simulink model "Aufgabe1_sim"  (R2023b)
settings: Solver=VariableStepAuto  StartTime=0.0  StopTime=1  RelTol=1e-3
values from neighbouring files (symbols this model uses):
  ci = 0.01    [Aufgabe1_param.m]
  cy = 1    [Aufgabe1_param.m]
  L = 0.1    [Aufgabe1_param.m]
  m = 10e-3    (= 0.01)    [Aufgabe1_param.m]
  R = 5    [Aufgabe1_param.m]
settings Model: Creator=rouven  LastModifiedBy=rouven

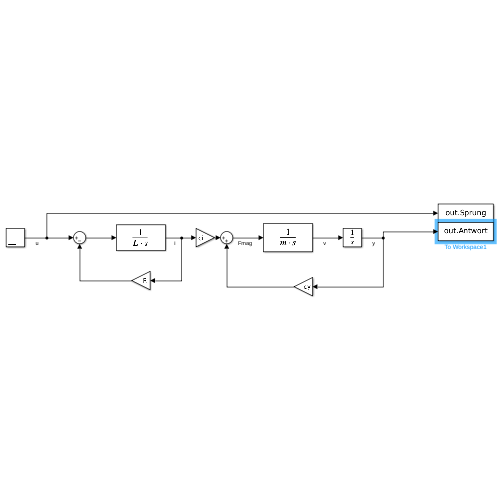
[thumbnail: Simulink's stored preview of the top-level diagram]
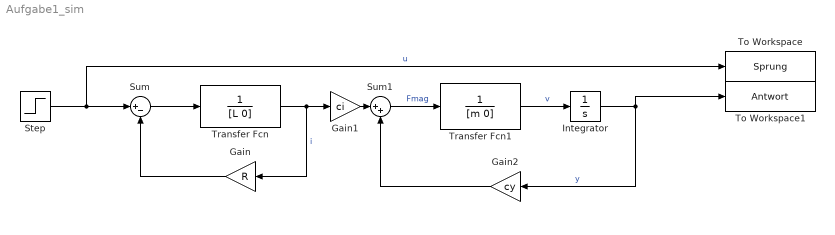
== system Aufgabe1_sim ==
  Gain : Gain  Gain=R
  Gain1 : Gain  Gain=ci
  Gain2 : Gain  Gain=cy
  Integrator : Integrator
  Step : Step  Time=0  SampleTime=0
  Sum : Sum  Inputs=|+-
  Sum1 : Sum  Inputs=|++
  To Workspace : ToWorkspace  VariableName=Sprung  SaveFormat=Timeseries  SampleTime=-1
  To Workspace1 : ToWorkspace  VariableName=Antwort  SaveFormat=Timeseries  SampleTime=-1
  Transfer Fcn : TransferFcn  Denominator=[L 0]
  Transfer Fcn1 : TransferFcn  Denominator=[m 0]
  wires:
  Sum/1 -> Transfer Fcn/1
  Gain/1 -> Sum/2
  Transfer Fcn/1 -> Gain/1, Gain1/1  "i"
  Gain1/1 -> Sum1/1
  Sum1/1 -> Transfer Fcn1/1  "Fmag"
  Transfer Fcn1/1 -> Integrator/1  "v"
  Integrator/1 -> To Workspace1/1, Gain2/1  "y"
  Gain2/1 -> Sum1/2
  Step/1 -> To Workspace/1, Sum/1  "u"
